simulink model "RADTRANS002"  (R2020b)
settings: Solver=VariableStepAuto  StartTime=0.0  StopTime=10.0  RelTol=1e-3
undefined symbols (not defined in the file): Line_110_C, Line_110_L, Line_110_R, Line_220_C, Line_220_L, Line_220_R, Line_35_C, Line_35_L, Line_35_R, Line_6_L, Line_6_R, Sys_f_Hz, Sys_V_net_kV, Tr_110_35_L_pu, Tr_110_35_R_pu, Tr_110_35_Sn_VA, Tr_110_35_V_HV_kV, Tr_110_35_V_LV_kV, Tr_110_6_L_pu, Tr_110_6_R_pu, Tr_110_6_Sn_VA, Tr_110_6_V_HV_kV, Tr_110_6_V_LV_kV, Tr_220_110_L_pu, Tr_220_110_R_pu, Tr_220_110_Sn_VA, Tr_220_110_V_HV_kV, Tr_220_110_V_LV_kV, Tr_35_04_L_pu, Tr_35_04_R_pu, Tr_35_04_Sn_VA, Tr_35_04_V_HV_kV, Tr_35_04_V_LV_kV, Tr_6_04_L_pu, Tr_6_04_R_pu, Tr_6_04_Sn_VA, Tr_6_04_V_HV_kV, Tr_6_04_V_LV_kV, Ts_powergui
libraries: dspstat3 x288, powerlib x202, powerlib_meascontrol x72
(part 3 of 7)

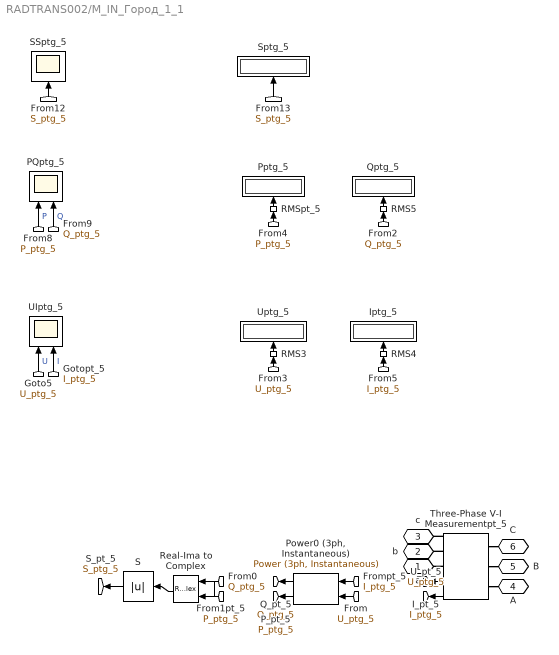
== system RADTRANS002/M_IN_Город_1_1 ==
  Iptg_5 : Display
      settings: Format=bank
  PQptg_5 : Scope  NumInputPorts=2
  "Power0 (3ph, Instantaneous)" : powerlib_meascontrol/Measurements/Power (3ph, Instantaneous)
  Pptg_5 : Display
      settings: Format=bank
  Qptg_5 : Display
      settings: Format=bank
  RMS3 : dspstat3/RMS  run=off  directionMode=Each column  dimension=1  InputProcessing=Columns as channels (frame based)  reset_popup=None
  RMS4 : dspstat3/RMS  run=off  directionMode=Each column  dimension=1  InputProcessing=Columns as channels (frame based)  reset_popup=None
  RMS5 : dspstat3/RMS  run=off  directionMode=Each column  dimension=1  InputProcessing=Columns as channels (frame based)  reset_popup=None
  RMSpt_5 : dspstat3/RMS  run=off  directionMode=Each column  dimension=1  InputProcessing=Columns as channels (frame based)  reset_popup=None
  Real-Ima to Complex : RealImagToComplex
  S : Abs
  SSptg_5 : Scope
  Sptg_5 : Display
      settings: Format=bank
  Three-Phase V-I Measurementpt_5 : powerlib/Measurements/Three-Phase V-I Measurement  VoltageMeasurement=phase-to-ground  SetLabelV=off  LabelV=Vabc  Vpu=off  VpuLL=off  CurrentMeasurement=yes  SetLabelI=off  LabelI=Iabc  Ipu=off  Pbase=100e6  Vbase=500e3  OutputType=Complex  PhasorSimulation=off  PSBequivalent=0
  UIptg_5 : Scope  NumInputPorts=2
  Uptg_5 : Display
      settings: Format=bank
  a : PMIOPort  Side=Right
  b : PMIOPort  Port=2  Side=Right
  c : PMIOPort  Port=3  Side=Right
  A : PMIOPort  Port=4  Side=Left
  B : PMIOPort  Port=5  Side=Left
  C : PMIOPort  Port=6  Side=Left
  tag scope: I_ptg_5=global, P_ptg_5=global, Q_ptg_5=global, S_ptg_5=global, U_ptg_5=global
  wires:
  S/1 -> [S_ptg_5]
  Real-Ima to Complex/1 -> S/1
  [S_ptg_5] -> Sptg_5/1
  [S_ptg_5] -> SSptg_5/1
  [P_ptg_5] -> RMSpt_5/1
  RMSpt_5/1 -> Pptg_5/1
  RMS5/1 -> Qptg_5/1
  [U_ptg_5] -> RMS3/1
  RMS3/1 -> Uptg_5/1
  [P_ptg_5] -> Real-Ima to Complex/1
  [Q_ptg_5] -> RMS5/1
  [I_ptg_5] -> RMS4/1
  RMS4/1 -> Iptg_5/1
  [U_ptg_5] -> UIptg_5/1  "U"
  [P_ptg_5] -> PQptg_5/1  "P"
  [I_ptg_5] -> UIptg_5/2  "I"
  Three-Phase V-I Measurementpt_5/1 -> [U_ptg_5]
  [Q_ptg_5] -> Real-Ima to Complex/2
  Three-Phase V-I Measurementpt_5/2 -> [I_ptg_5]
  [U_ptg_5] -> "Power0 (3ph, Instantaneous)"/1
  [I_ptg_5] -> "Power0 (3ph, Instantaneous)"/2
  "Power0 (3ph, Instantaneous)"/2 -> [Q_ptg_5]
  "Power0 (3ph, Instantaneous)"/1 -> [P_ptg_5]
  [Q_ptg_5] -> PQptg_5/2  "Q"
  connections:
  Three-Phase V-I Measurementpt_5/LConn1 -- A/RConn1
  Three-Phase V-I Measurementpt_5/RConn1 -- a/RConn1
  Three-Phase V-I Measurementpt_5/LConn2 -- B/RConn1
  Three-Phase V-I Measurementpt_5/LConn3 -- C/RConn1
  Three-Phase V-I Measurementpt_5/RConn3 -- c/RConn1
  Three-Phase V-I Measurementpt_5/RConn2 -- b/RConn1

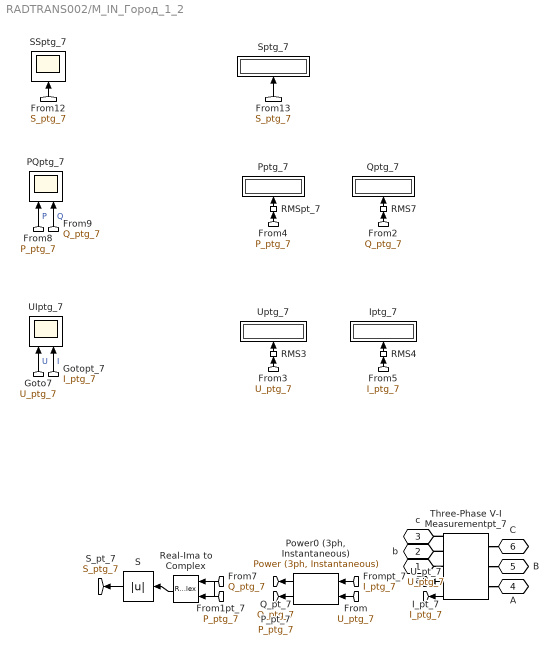
== system RADTRANS002/M_IN_Город_1_2 ==
  Iptg_7 : Display
      settings: Format=bank
  PQptg_7 : Scope  NumInputPorts=2
  "Power0 (3ph, Instantaneous)" : powerlib_meascontrol/Measurements/Power (3ph, Instantaneous)
  Pptg_7 : Display
      settings: Format=bank
  Qptg_7 : Display
      settings: Format=bank
  RMS3 : dspstat3/RMS  run=off  directionMode=Each column  dimension=1  InputProcessing=Columns as channels (frame based)  reset_popup=None
  RMS4 : dspstat3/RMS  run=off  directionMode=Each column  dimension=1  InputProcessing=Columns as channels (frame based)  reset_popup=None
  RMS7 : dspstat3/RMS  run=off  directionMode=Each column  dimension=1  InputProcessing=Columns as channels (frame based)  reset_popup=None
  RMSpt_7 : dspstat3/RMS  run=off  directionMode=Each column  dimension=1  InputProcessing=Columns as channels (frame based)  reset_popup=None
  Real-Ima to Complex : RealImagToComplex
  S : Abs
  SSptg_7 : Scope
  Sptg_7 : Display
      settings: Format=bank
  Three-Phase V-I Measurementpt_7 : powerlib/Measurements/Three-Phase V-I Measurement  VoltageMeasurement=phase-to-ground  SetLabelV=off  LabelV=Vabc  Vpu=off  VpuLL=off  CurrentMeasurement=yes  SetLabelI=off  LabelI=Iabc  Ipu=off  Pbase=100e6  Vbase=500e3  OutputType=Complex  PhasorSimulation=off  PSBequivalent=0
  UIptg_7 : Scope  NumInputPorts=2
  Uptg_7 : Display
      settings: Format=bank
  a : PMIOPort  Side=Right
  b : PMIOPort  Port=2  Side=Right
  c : PMIOPort  Port=3  Side=Right
  A : PMIOPort  Port=4  Side=Left
  B : PMIOPort  Port=5  Side=Left
  C : PMIOPort  Port=6  Side=Left
  tag scope: I_ptg_7=global, P_ptg_7=global, Q_ptg_7=global, S_ptg_7=global, U_ptg_7=global
  wires:
  S/1 -> [S_ptg_7]
  Real-Ima to Complex/1 -> S/1
  [S_ptg_7] -> Sptg_7/1
  [S_ptg_7] -> SSptg_7/1
  [P_ptg_7] -> RMSpt_7/1
  RMSpt_7/1 -> Pptg_7/1
  RMS7/1 -> Qptg_7/1
  [U_ptg_7] -> RMS3/1
  RMS3/1 -> Uptg_7/1
  [P_ptg_7] -> Real-Ima to Complex/1
  [Q_ptg_7] -> RMS7/1
  [I_ptg_7] -> RMS4/1
  RMS4/1 -> Iptg_7/1
  [U_ptg_7] -> UIptg_7/1  "U"
  [P_ptg_7] -> PQptg_7/1  "P"
  [I_ptg_7] -> UIptg_7/2  "I"
  Three-Phase V-I Measurementpt_7/1 -> [U_ptg_7]
  [Q_ptg_7] -> Real-Ima to Complex/2
  Three-Phase V-I Measurementpt_7/2 -> [I_ptg_7]
  [U_ptg_7] -> "Power0 (3ph, Instantaneous)"/1
  [I_ptg_7] -> "Power0 (3ph, Instantaneous)"/2
  "Power0 (3ph, Instantaneous)"/2 -> [Q_ptg_7]
  "Power0 (3ph, Instantaneous)"/1 -> [P_ptg_7]
  [Q_ptg_7] -> PQptg_7/2  "Q"
  connections:
  Three-Phase V-I Measurementpt_7/LConn1 -- A/RConn1
  Three-Phase V-I Measurementpt_7/RConn1 -- a/RConn1
  Three-Phase V-I Measurementpt_7/LConn2 -- B/RConn1
  Three-Phase V-I Measurementpt_7/LConn3 -- C/RConn1
  Three-Phase V-I Measurementpt_7/RConn3 -- c/RConn1
  Three-Phase V-I Measurementpt_7/RConn2 -- b/RConn1

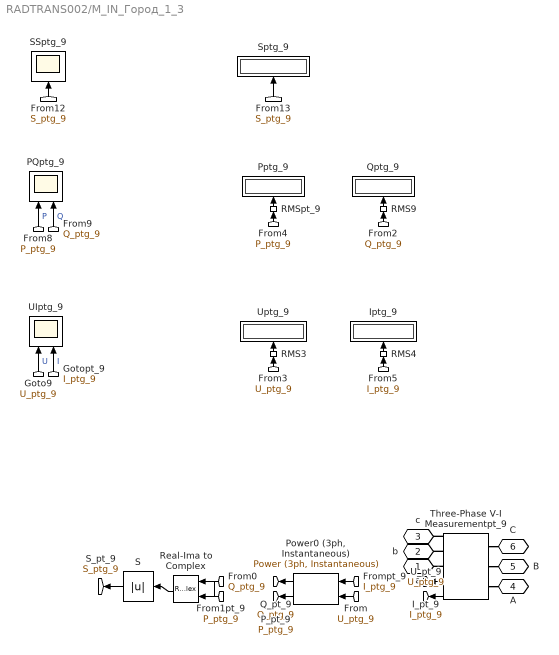
== system RADTRANS002/M_IN_Город_1_3 ==
  Iptg_9 : Display
      settings: Format=bank
  PQptg_9 : Scope  NumInputPorts=2
  "Power0 (3ph, Instantaneous)" : powerlib_meascontrol/Measurements/Power (3ph, Instantaneous)
  Pptg_9 : Display
      settings: Format=bank
  Qptg_9 : Display
      settings: Format=bank
  RMS3 : dspstat3/RMS  run=off  directionMode=Each column  dimension=1  InputProcessing=Columns as channels (frame based)  reset_popup=None
  RMS4 : dspstat3/RMS  run=off  directionMode=Each column  dimension=1  InputProcessing=Columns as channels (frame based)  reset_popup=None
  RMS9 : dspstat3/RMS  run=off  directionMode=Each column  dimension=1  InputProcessing=Columns as channels (frame based)  reset_popup=None
  RMSpt_9 : dspstat3/RMS  run=off  directionMode=Each column  dimension=1  InputProcessing=Columns as channels (frame based)  reset_popup=None
  Real-Ima to Complex : RealImagToComplex
  S : Abs
  SSptg_9 : Scope
  Sptg_9 : Display
      settings: Format=bank
  Three-Phase V-I Measurementpt_9 : powerlib/Measurements/Three-Phase V-I Measurement  VoltageMeasurement=phase-to-ground  SetLabelV=off  LabelV=Vabc  Vpu=off  VpuLL=off  CurrentMeasurement=yes  SetLabelI=off  LabelI=Iabc  Ipu=off  Pbase=100e6  Vbase=500e3  OutputType=Complex  PhasorSimulation=off  PSBequivalent=0
  UIptg_9 : Scope  NumInputPorts=2
  Uptg_9 : Display
      settings: Format=bank
  a : PMIOPort  Side=Right
  b : PMIOPort  Port=2  Side=Right
  c : PMIOPort  Port=3  Side=Right
  A : PMIOPort  Port=4  Side=Left
  B : PMIOPort  Port=5  Side=Left
  C : PMIOPort  Port=6  Side=Left
  tag scope: I_ptg_9=global, P_ptg_9=global, Q_ptg_9=global, S_ptg_9=global, U_ptg_9=global
  wires:
  S/1 -> [S_ptg_9]
  Real-Ima to Complex/1 -> S/1
  [S_ptg_9] -> Sptg_9/1
  [S_ptg_9] -> SSptg_9/1
  [P_ptg_9] -> RMSpt_9/1
  RMSpt_9/1 -> Pptg_9/1
  RMS9/1 -> Qptg_9/1
  [U_ptg_9] -> RMS3/1
  RMS3/1 -> Uptg_9/1
  [P_ptg_9] -> Real-Ima to Complex/1
  [Q_ptg_9] -> RMS9/1
  [I_ptg_9] -> RMS4/1
  RMS4/1 -> Iptg_9/1
  [U_ptg_9] -> UIptg_9/1  "U"
  [P_ptg_9] -> PQptg_9/1  "P"
  [I_ptg_9] -> UIptg_9/2  "I"
  Three-Phase V-I Measurementpt_9/1 -> [U_ptg_9]
  [Q_ptg_9] -> Real-Ima to Complex/2
  Three-Phase V-I Measurementpt_9/2 -> [I_ptg_9]
  [U_ptg_9] -> "Power0 (3ph, Instantaneous)"/1
  [I_ptg_9] -> "Power0 (3ph, Instantaneous)"/2
  "Power0 (3ph, Instantaneous)"/2 -> [Q_ptg_9]
  "Power0 (3ph, Instantaneous)"/1 -> [P_ptg_9]
  [Q_ptg_9] -> PQptg_9/2  "Q"
  connections:
  Three-Phase V-I Measurementpt_9/LConn1 -- A/RConn1
  Three-Phase V-I Measurementpt_9/RConn1 -- a/RConn1
  Three-Phase V-I Measurementpt_9/LConn2 -- B/RConn1
  Three-Phase V-I Measurementpt_9/LConn3 -- C/RConn1
  Three-Phase V-I Measurementpt_9/RConn3 -- c/RConn1
  Three-Phase V-I Measurementpt_9/RConn2 -- b/RConn1

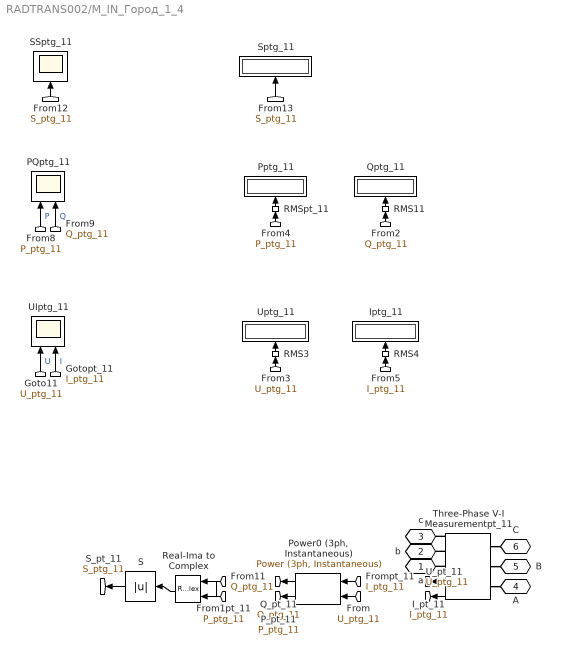
== system RADTRANS002/M_IN_Город_1_4 ==
  Iptg_11 : Display
      settings: Format=bank
  PQptg_11 : Scope  NumInputPorts=2
  "Power0 (3ph, Instantaneous)" : powerlib_meascontrol/Measurements/Power (3ph, Instantaneous)
  Pptg_11 : Display
      settings: Format=bank
  Qptg_11 : Display
      settings: Format=bank
  RMS11 : dspstat3/RMS  run=off  directionMode=Each column  dimension=1  InputProcessing=Columns as channels (frame based)  reset_popup=None
  RMS3 : dspstat3/RMS  run=off  directionMode=Each column  dimension=1  InputProcessing=Columns as channels (frame based)  reset_popup=None
  RMS4 : dspstat3/RMS  run=off  directionMode=Each column  dimension=1  InputProcessing=Columns as channels (frame based)  reset_popup=None
  RMSpt_11 : dspstat3/RMS  run=off  directionMode=Each column  dimension=1  InputProcessing=Columns as channels (frame based)  reset_popup=None
  Real-Ima to Complex : RealImagToComplex
  S : Abs
  SSptg_11 : Scope
  Sptg_11 : Display
      settings: Format=bank
  Three-Phase V-I Measurementpt_11 : powerlib/Measurements/Three-Phase V-I Measurement  VoltageMeasurement=phase-to-ground  SetLabelV=off  LabelV=Vabc  Vpu=off  VpuLL=off  CurrentMeasurement=yes  SetLabelI=off  LabelI=Iabc  Ipu=off  Pbase=100e6  Vbase=500e3  OutputType=Complex  PhasorSimulation=off  PSBequivalent=0
  UIptg_11 : Scope  NumInputPorts=2
  Uptg_11 : Display
      settings: Format=bank
  a : PMIOPort  Side=Right
  b : PMIOPort  Port=2  Side=Right
  c : PMIOPort  Port=3  Side=Right
  A : PMIOPort  Port=4  Side=Left
  B : PMIOPort  Port=5  Side=Left
  C : PMIOPort  Port=6  Side=Left
  tag scope: I_ptg_11=global, P_ptg_11=global, Q_ptg_11=global, S_ptg_11=global, U_ptg_11=global
  wires:
  S/1 -> [S_ptg_11]
  Real-Ima to Complex/1 -> S/1
  [S_ptg_11] -> Sptg_11/1
  [S_ptg_11] -> SSptg_11/1
  [P_ptg_11] -> RMSpt_11/1
  RMSpt_11/1 -> Pptg_11/1
  RMS11/1 -> Qptg_11/1
  [U_ptg_11] -> RMS3/1
  RMS3/1 -> Uptg_11/1
  [P_ptg_11] -> Real-Ima to Complex/1
  [Q_ptg_11] -> RMS11/1
  [I_ptg_11] -> RMS4/1
  RMS4/1 -> Iptg_11/1
  [U_ptg_11] -> UIptg_11/1  "U"
  [P_ptg_11] -> PQptg_11/1  "P"
  [I_ptg_11] -> UIptg_11/2  "I"
  Three-Phase V-I Measurementpt_11/1 -> [U_ptg_11]
  [Q_ptg_11] -> Real-Ima to Complex/2
  Three-Phase V-I Measurementpt_11/2 -> [I_ptg_11]
  [U_ptg_11] -> "Power0 (3ph, Instantaneous)"/1
  [I_ptg_11] -> "Power0 (3ph, Instantaneous)"/2
  "Power0 (3ph, Instantaneous)"/2 -> [Q_ptg_11]
  "Power0 (3ph, Instantaneous)"/1 -> [P_ptg_11]
  [Q_ptg_11] -> PQptg_11/2  "Q"
  connections:
  Three-Phase V-I Measurementpt_11/LConn1 -- A/RConn1
  Three-Phase V-I Measurementpt_11/RConn1 -- a/RConn1
  Three-Phase V-I Measurementpt_11/LConn2 -- B/RConn1
  Three-Phase V-I Measurementpt_11/LConn3 -- C/RConn1
  Three-Phase V-I Measurementpt_11/RConn3 -- c/RConn1
  Three-Phase V-I Measurementpt_11/RConn2 -- b/RConn1

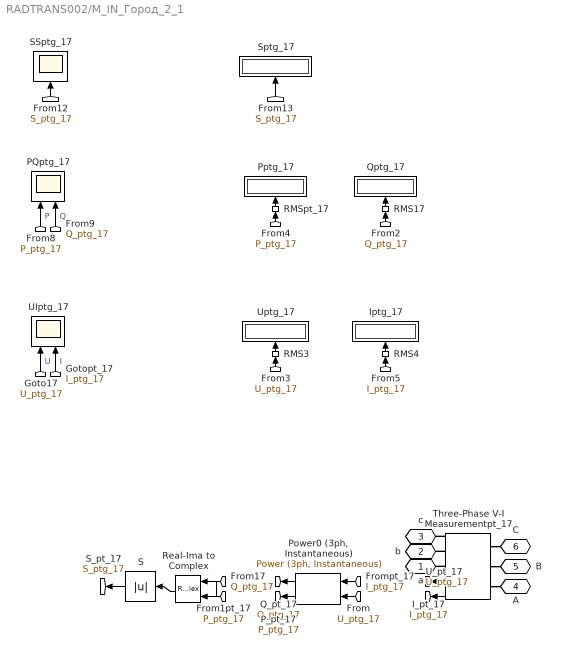
== system RADTRANS002/M_IN_Город_2_1 ==
  Iptg_17 : Display
      settings: Format=bank
  PQptg_17 : Scope  NumInputPorts=2
  "Power0 (3ph, Instantaneous)" : powerlib_meascontrol/Measurements/Power (3ph, Instantaneous)
  Pptg_17 : Display
      settings: Format=bank
  Qptg_17 : Display
      settings: Format=bank
  RMS17 : dspstat3/RMS  run=off  directionMode=Each column  dimension=1  InputProcessing=Columns as channels (frame based)  reset_popup=None
  RMS3 : dspstat3/RMS  run=off  directionMode=Each column  dimension=1  InputProcessing=Columns as channels (frame based)  reset_popup=None
  RMS4 : dspstat3/RMS  run=off  directionMode=Each column  dimension=1  InputProcessing=Columns as channels (frame based)  reset_popup=None
  RMSpt_17 : dspstat3/RMS  run=off  directionMode=Each column  dimension=1  InputProcessing=Columns as channels (frame based)  reset_popup=None
  Real-Ima to Complex : RealImagToComplex
  S : Abs
  SSptg_17 : Scope
  Sptg_17 : Display
      settings: Format=bank
  Three-Phase V-I Measurementpt_17 : powerlib/Measurements/Three-Phase V-I Measurement  VoltageMeasurement=phase-to-ground  SetLabelV=off  LabelV=Vabc  Vpu=off  VpuLL=off  CurrentMeasurement=yes  SetLabelI=off  LabelI=Iabc  Ipu=off  Pbase=100e6  Vbase=500e3  OutputType=Complex  PhasorSimulation=off  PSBequivalent=0
  UIptg_17 : Scope  NumInputPorts=2
  Uptg_17 : Display
      settings: Format=bank
  a : PMIOPort  Side=Right
  b : PMIOPort  Port=2  Side=Right
  c : PMIOPort  Port=3  Side=Right
  A : PMIOPort  Port=4  Side=Left
  B : PMIOPort  Port=5  Side=Left
  C : PMIOPort  Port=6  Side=Left
  tag scope: I_ptg_17=global, P_ptg_17=global, Q_ptg_17=global, S_ptg_17=global, U_ptg_17=global
  wires:
  S/1 -> [S_ptg_17]
  Real-Ima to Complex/1 -> S/1
  [S_ptg_17] -> Sptg_17/1
  [S_ptg_17] -> SSptg_17/1
  [P_ptg_17] -> RMSpt_17/1
  RMSpt_17/1 -> Pptg_17/1
  RMS17/1 -> Qptg_17/1
  [U_ptg_17] -> RMS3/1
  RMS3/1 -> Uptg_17/1
  [P_ptg_17] -> Real-Ima to Complex/1
  [Q_ptg_17] -> RMS17/1
  [I_ptg_17] -> RMS4/1
  RMS4/1 -> Iptg_17/1
  [U_ptg_17] -> UIptg_17/1  "U"
  [P_ptg_17] -> PQptg_17/1  "P"
  [I_ptg_17] -> UIptg_17/2  "I"
  Three-Phase V-I Measurementpt_17/1 -> [U_ptg_17]
  [Q_ptg_17] -> Real-Ima to Complex/2
  Three-Phase V-I Measurementpt_17/2 -> [I_ptg_17]
  [U_ptg_17] -> "Power0 (3ph, Instantaneous)"/1
  [I_ptg_17] -> "Power0 (3ph, Instantaneous)"/2
  "Power0 (3ph, Instantaneous)"/2 -> [Q_ptg_17]
  "Power0 (3ph, Instantaneous)"/1 -> [P_ptg_17]
  [Q_ptg_17] -> PQptg_17/2  "Q"
  connections:
  Three-Phase V-I Measurementpt_17/LConn1 -- A/RConn1
  Three-Phase V-I Measurementpt_17/RConn1 -- a/RConn1
  Three-Phase V-I Measurementpt_17/LConn2 -- B/RConn1
  Three-Phase V-I Measurementpt_17/LConn3 -- C/RConn1
  Three-Phase V-I Measurementpt_17/RConn3 -- c/RConn1
  Three-Phase V-I Measurementpt_17/RConn2 -- b/RConn1

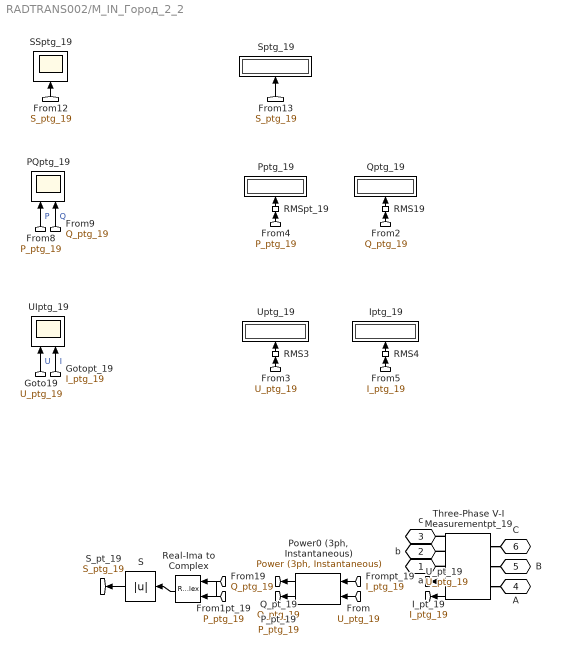
== system RADTRANS002/M_IN_Город_2_2 ==
  Iptg_19 : Display
      settings: Format=bank
  PQptg_19 : Scope  NumInputPorts=2
  "Power0 (3ph, Instantaneous)" : powerlib_meascontrol/Measurements/Power (3ph, Instantaneous)
  Pptg_19 : Display
      settings: Format=bank
  Qptg_19 : Display
      settings: Format=bank
  RMS19 : dspstat3/RMS  run=off  directionMode=Each column  dimension=1  InputProcessing=Columns as channels (frame based)  reset_popup=None
  RMS3 : dspstat3/RMS  run=off  directionMode=Each column  dimension=1  InputProcessing=Columns as channels (frame based)  reset_popup=None
  RMS4 : dspstat3/RMS  run=off  directionMode=Each column  dimension=1  InputProcessing=Columns as channels (frame based)  reset_popup=None
  RMSpt_19 : dspstat3/RMS  run=off  directionMode=Each column  dimension=1  InputProcessing=Columns as channels (frame based)  reset_popup=None
  Real-Ima to Complex : RealImagToComplex
  S : Abs
  SSptg_19 : Scope
  Sptg_19 : Display
      settings: Format=bank
  Three-Phase V-I Measurementpt_19 : powerlib/Measurements/Three-Phase V-I Measurement  VoltageMeasurement=phase-to-ground  SetLabelV=off  LabelV=Vabc  Vpu=off  VpuLL=off  CurrentMeasurement=yes  SetLabelI=off  LabelI=Iabc  Ipu=off  Pbase=100e6  Vbase=500e3  OutputType=Complex  PhasorSimulation=off  PSBequivalent=0
  UIptg_19 : Scope  NumInputPorts=2
  Uptg_19 : Display
      settings: Format=bank
  a : PMIOPort  Side=Right
  b : PMIOPort  Port=2  Side=Right
  c : PMIOPort  Port=3  Side=Right
  A : PMIOPort  Port=4  Side=Left
  B : PMIOPort  Port=5  Side=Left
  C : PMIOPort  Port=6  Side=Left
  tag scope: I_ptg_19=global, P_ptg_19=global, Q_ptg_19=global, S_ptg_19=global, U_ptg_19=global
  wires:
  S/1 -> [S_ptg_19]
  Real-Ima to Complex/1 -> S/1
  [S_ptg_19] -> Sptg_19/1
  [S_ptg_19] -> SSptg_19/1
  [P_ptg_19] -> RMSpt_19/1
  RMSpt_19/1 -> Pptg_19/1
  RMS19/1 -> Qptg_19/1
  [U_ptg_19] -> RMS3/1
  RMS3/1 -> Uptg_19/1
  [P_ptg_19] -> Real-Ima to Complex/1
  [Q_ptg_19] -> RMS19/1
  [I_ptg_19] -> RMS4/1
  RMS4/1 -> Iptg_19/1
  [U_ptg_19] -> UIptg_19/1  "U"
  [P_ptg_19] -> PQptg_19/1  "P"
  [I_ptg_19] -> UIptg_19/2  "I"
  Three-Phase V-I Measurementpt_19/1 -> [U_ptg_19]
  [Q_ptg_19] -> Real-Ima to Complex/2
  Three-Phase V-I Measurementpt_19/2 -> [I_ptg_19]
  [U_ptg_19] -> "Power0 (3ph, Instantaneous)"/1
  [I_ptg_19] -> "Power0 (3ph, Instantaneous)"/2
  "Power0 (3ph, Instantaneous)"/2 -> [Q_ptg_19]
  "Power0 (3ph, Instantaneous)"/1 -> [P_ptg_19]
  [Q_ptg_19] -> PQptg_19/2  "Q"
  connections:
  Three-Phase V-I Measurementpt_19/LConn1 -- A/RConn1
  Three-Phase V-I Measurementpt_19/RConn1 -- a/RConn1
  Three-Phase V-I Measurementpt_19/LConn2 -- B/RConn1
  Three-Phase V-I Measurementpt_19/LConn3 -- C/RConn1
  Three-Phase V-I Measurementpt_19/RConn3 -- c/RConn1
  Three-Phase V-I Measurementpt_19/RConn2 -- b/RConn1

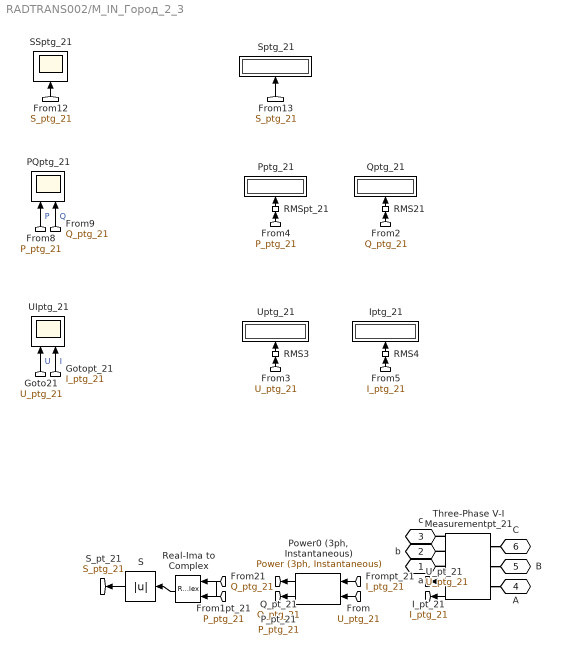
== system RADTRANS002/M_IN_Город_2_3 ==
  Iptg_21 : Display
      settings: Format=bank
  PQptg_21 : Scope  NumInputPorts=2
  "Power0 (3ph, Instantaneous)" : powerlib_meascontrol/Measurements/Power (3ph, Instantaneous)
  Pptg_21 : Display
      settings: Format=bank
  Qptg_21 : Display
      settings: Format=bank
  RMS21 : dspstat3/RMS  run=off  directionMode=Each column  dimension=1  InputProcessing=Columns as channels (frame based)  reset_popup=None
  RMS3 : dspstat3/RMS  run=off  directionMode=Each column  dimension=1  InputProcessing=Columns as channels (frame based)  reset_popup=None
  RMS4 : dspstat3/RMS  run=off  directionMode=Each column  dimension=1  InputProcessing=Columns as channels (frame based)  reset_popup=None
  RMSpt_21 : dspstat3/RMS  run=off  directionMode=Each column  dimension=1  InputProcessing=Columns as channels (frame based)  reset_popup=None
  Real-Ima to Complex : RealImagToComplex
  S : Abs
  SSptg_21 : Scope
  Sptg_21 : Display
      settings: Format=bank
  Three-Phase V-I Measurementpt_21 : powerlib/Measurements/Three-Phase V-I Measurement  VoltageMeasurement=phase-to-ground  SetLabelV=off  LabelV=Vabc  Vpu=off  VpuLL=off  CurrentMeasurement=yes  SetLabelI=off  LabelI=Iabc  Ipu=off  Pbase=100e6  Vbase=500e3  OutputType=Complex  PhasorSimulation=off  PSBequivalent=0
  UIptg_21 : Scope  NumInputPorts=2
  Uptg_21 : Display
      settings: Format=bank
  a : PMIOPort  Side=Right
  b : PMIOPort  Port=2  Side=Right
  c : PMIOPort  Port=3  Side=Right
  A : PMIOPort  Port=4  Side=Left
  B : PMIOPort  Port=5  Side=Left
  C : PMIOPort  Port=6  Side=Left
  tag scope: I_ptg_21=global, P_ptg_21=global, Q_ptg_21=global, S_ptg_21=global, U_ptg_21=global
  wires:
  S/1 -> [S_ptg_21]
  Real-Ima to Complex/1 -> S/1
  [S_ptg_21] -> Sptg_21/1
  [S_ptg_21] -> SSptg_21/1
  [P_ptg_21] -> RMSpt_21/1
  RMSpt_21/1 -> Pptg_21/1
  RMS21/1 -> Qptg_21/1
  [U_ptg_21] -> RMS3/1
  RMS3/1 -> Uptg_21/1
  [P_ptg_21] -> Real-Ima to Complex/1
  [Q_ptg_21] -> RMS21/1
  [I_ptg_21] -> RMS4/1
  RMS4/1 -> Iptg_21/1
  [U_ptg_21] -> UIptg_21/1  "U"
  [P_ptg_21] -> PQptg_21/1  "P"
  [I_ptg_21] -> UIptg_21/2  "I"
  Three-Phase V-I Measurementpt_21/1 -> [U_ptg_21]
  [Q_ptg_21] -> Real-Ima to Complex/2
  Three-Phase V-I Measurementpt_21/2 -> [I_ptg_21]
  [U_ptg_21] -> "Power0 (3ph, Instantaneous)"/1
  [I_ptg_21] -> "Power0 (3ph, Instantaneous)"/2
  "Power0 (3ph, Instantaneous)"/2 -> [Q_ptg_21]
  "Power0 (3ph, Instantaneous)"/1 -> [P_ptg_21]
  [Q_ptg_21] -> PQptg_21/2  "Q"
  connections:
  Three-Phase V-I Measurementpt_21/LConn1 -- A/RConn1
  Three-Phase V-I Measurementpt_21/RConn1 -- a/RConn1
  Three-Phase V-I Measurementpt_21/LConn2 -- B/RConn1
  Three-Phase V-I Measurementpt_21/LConn3 -- C/RConn1
  Three-Phase V-I Measurementpt_21/RConn3 -- c/RConn1
  Three-Phase V-I Measurementpt_21/RConn2 -- b/RConn1

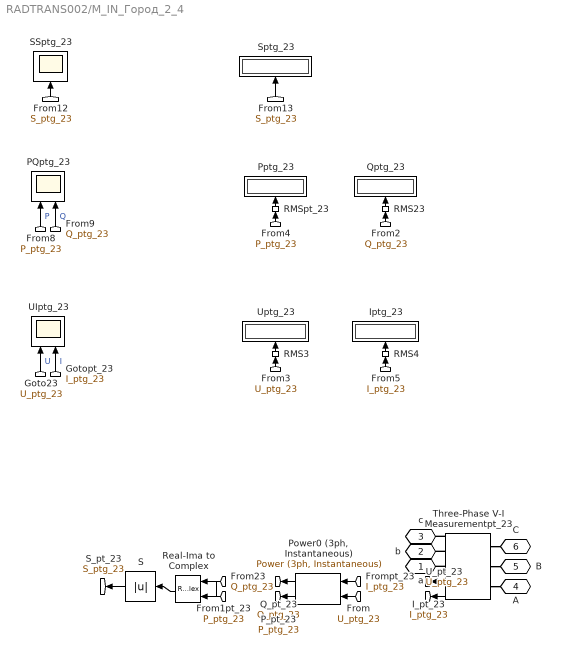
== system RADTRANS002/M_IN_Город_2_4 ==
  Iptg_23 : Display
      settings: Format=bank
  PQptg_23 : Scope  NumInputPorts=2
  "Power0 (3ph, Instantaneous)" : powerlib_meascontrol/Measurements/Power (3ph, Instantaneous)
  Pptg_23 : Display
      settings: Format=bank
  Qptg_23 : Display
      settings: Format=bank
  RMS23 : dspstat3/RMS  run=off  directionMode=Each column  dimension=1  InputProcessing=Columns as channels (frame based)  reset_popup=None
  RMS3 : dspstat3/RMS  run=off  directionMode=Each column  dimension=1  InputProcessing=Columns as channels (frame based)  reset_popup=None
  RMS4 : dspstat3/RMS  run=off  directionMode=Each column  dimension=1  InputProcessing=Columns as channels (frame based)  reset_popup=None
  RMSpt_23 : dspstat3/RMS  run=off  directionMode=Each column  dimension=1  InputProcessing=Columns as channels (frame based)  reset_popup=None
  Real-Ima to Complex : RealImagToComplex
  S : Abs
  SSptg_23 : Scope
  Sptg_23 : Display
      settings: Format=bank
  Three-Phase V-I Measurementpt_23 : powerlib/Measurements/Three-Phase V-I Measurement  VoltageMeasurement=phase-to-ground  SetLabelV=off  LabelV=Vabc  Vpu=off  VpuLL=off  CurrentMeasurement=yes  SetLabelI=off  LabelI=Iabc  Ipu=off  Pbase=100e6  Vbase=500e3  OutputType=Complex  PhasorSimulation=off  PSBequivalent=0
  UIptg_23 : Scope  NumInputPorts=2
  Uptg_23 : Display
      settings: Format=bank
  a : PMIOPort  Side=Right
  b : PMIOPort  Port=2  Side=Right
  c : PMIOPort  Port=3  Side=Right
  A : PMIOPort  Port=4  Side=Left
  B : PMIOPort  Port=5  Side=Left
  C : PMIOPort  Port=6  Side=Left
  tag scope: I_ptg_23=global, P_ptg_23=global, Q_ptg_23=global, S_ptg_23=global, U_ptg_23=global
  wires:
  S/1 -> [S_ptg_23]
  Real-Ima to Complex/1 -> S/1
  [S_ptg_23] -> Sptg_23/1
  [S_ptg_23] -> SSptg_23/1
  [P_ptg_23] -> RMSpt_23/1
  RMSpt_23/1 -> Pptg_23/1
  RMS23/1 -> Qptg_23/1
  [U_ptg_23] -> RMS3/1
  RMS3/1 -> Uptg_23/1
  [P_ptg_23] -> Real-Ima to Complex/1
  [Q_ptg_23] -> RMS23/1
  [I_ptg_23] -> RMS4/1
  RMS4/1 -> Iptg_23/1
  [U_ptg_23] -> UIptg_23/1  "U"
  [P_ptg_23] -> PQptg_23/1  "P"
  [I_ptg_23] -> UIptg_23/2  "I"
  Three-Phase V-I Measurementpt_23/1 -> [U_ptg_23]
  [Q_ptg_23] -> Real-Ima to Complex/2
  Three-Phase V-I Measurementpt_23/2 -> [I_ptg_23]
  [U_ptg_23] -> "Power0 (3ph, Instantaneous)"/1
  [I_ptg_23] -> "Power0 (3ph, Instantaneous)"/2
  "Power0 (3ph, Instantaneous)"/2 -> [Q_ptg_23]
  "Power0 (3ph, Instantaneous)"/1 -> [P_ptg_23]
  [Q_ptg_23] -> PQptg_23/2  "Q"
  connections:
  Three-Phase V-I Measurementpt_23/LConn1 -- A/RConn1
  Three-Phase V-I Measurementpt_23/RConn1 -- a/RConn1
  Three-Phase V-I Measurementpt_23/LConn2 -- B/RConn1
  Three-Phase V-I Measurementpt_23/LConn3 -- C/RConn1
  Three-Phase V-I Measurementpt_23/RConn3 -- c/RConn1
  Three-Phase V-I Measurementpt_23/RConn2 -- b/RConn1

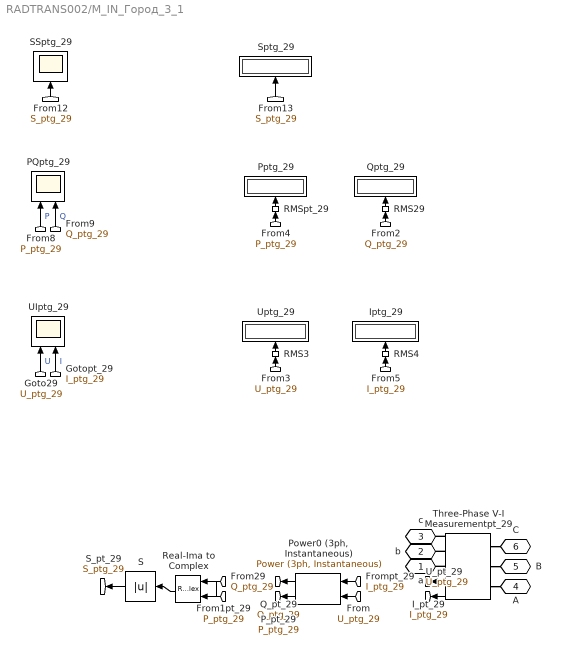
== system RADTRANS002/M_IN_Город_3_1 ==
  Iptg_29 : Display
      settings: Format=bank
  PQptg_29 : Scope  NumInputPorts=2
  "Power0 (3ph, Instantaneous)" : powerlib_meascontrol/Measurements/Power (3ph, Instantaneous)
  Pptg_29 : Display
      settings: Format=bank
  Qptg_29 : Display
      settings: Format=bank
  RMS29 : dspstat3/RMS  run=off  directionMode=Each column  dimension=1  InputProcessing=Columns as channels (frame based)  reset_popup=None
  RMS3 : dspstat3/RMS  run=off  directionMode=Each column  dimension=1  InputProcessing=Columns as channels (frame based)  reset_popup=None
  RMS4 : dspstat3/RMS  run=off  directionMode=Each column  dimension=1  InputProcessing=Columns as channels (frame based)  reset_popup=None
  RMSpt_29 : dspstat3/RMS  run=off  directionMode=Each column  dimension=1  InputProcessing=Columns as channels (frame based)  reset_popup=None
  Real-Ima to Complex : RealImagToComplex
  S : Abs
  SSptg_29 : Scope
  Sptg_29 : Display
      settings: Format=bank
  Three-Phase V-I Measurementpt_29 : powerlib/Measurements/Three-Phase V-I Measurement  VoltageMeasurement=phase-to-ground  SetLabelV=off  LabelV=Vabc  Vpu=off  VpuLL=off  CurrentMeasurement=yes  SetLabelI=off  LabelI=Iabc  Ipu=off  Pbase=100e6  Vbase=500e3  OutputType=Complex  PhasorSimulation=off  PSBequivalent=0
  UIptg_29 : Scope  NumInputPorts=2
  Uptg_29 : Display
      settings: Format=bank
  a : PMIOPort  Side=Right
  b : PMIOPort  Port=2  Side=Right
  c : PMIOPort  Port=3  Side=Right
  A : PMIOPort  Port=4  Side=Left
  B : PMIOPort  Port=5  Side=Left
  C : PMIOPort  Port=6  Side=Left
  tag scope: I_ptg_29=global, P_ptg_29=global, Q_ptg_29=global, S_ptg_29=global, U_ptg_29=global
  wires:
  S/1 -> [S_ptg_29]
  Real-Ima to Complex/1 -> S/1
  [S_ptg_29] -> Sptg_29/1
  [S_ptg_29] -> SSptg_29/1
  [P_ptg_29] -> RMSpt_29/1
  RMSpt_29/1 -> Pptg_29/1
  RMS29/1 -> Qptg_29/1
  [U_ptg_29] -> RMS3/1
  RMS3/1 -> Uptg_29/1
  [P_ptg_29] -> Real-Ima to Complex/1
  [Q_ptg_29] -> RMS29/1
  [I_ptg_29] -> RMS4/1
  RMS4/1 -> Iptg_29/1
  [U_ptg_29] -> UIptg_29/1  "U"
  [P_ptg_29] -> PQptg_29/1  "P"
  [I_ptg_29] -> UIptg_29/2  "I"
  Three-Phase V-I Measurementpt_29/1 -> [U_ptg_29]
  [Q_ptg_29] -> Real-Ima to Complex/2
  Three-Phase V-I Measurementpt_29/2 -> [I_ptg_29]
  [U_ptg_29] -> "Power0 (3ph, Instantaneous)"/1
  [I_ptg_29] -> "Power0 (3ph, Instantaneous)"/2
  "Power0 (3ph, Instantaneous)"/2 -> [Q_ptg_29]
  "Power0 (3ph, Instantaneous)"/1 -> [P_ptg_29]
  [Q_ptg_29] -> PQptg_29/2  "Q"
  connections:
  Three-Phase V-I Measurementpt_29/LConn1 -- A/RConn1
  Three-Phase V-I Measurementpt_29/RConn1 -- a/RConn1
  Three-Phase V-I Measurementpt_29/LConn2 -- B/RConn1
  Three-Phase V-I Measurementpt_29/LConn3 -- C/RConn1
  Three-Phase V-I Measurementpt_29/RConn3 -- c/RConn1
  Three-Phase V-I Measurementpt_29/RConn2 -- b/RConn1

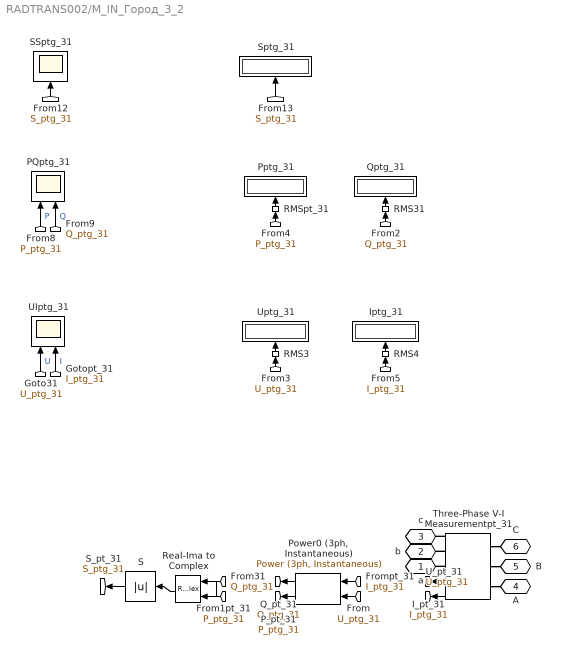
== system RADTRANS002/M_IN_Город_3_2 ==
  Iptg_31 : Display
      settings: Format=bank
  PQptg_31 : Scope  NumInputPorts=2
  "Power0 (3ph, Instantaneous)" : powerlib_meascontrol/Measurements/Power (3ph, Instantaneous)
  Pptg_31 : Display
      settings: Format=bank
  Qptg_31 : Display
      settings: Format=bank
  RMS3 : dspstat3/RMS  run=off  directionMode=Each column  dimension=1  InputProcessing=Columns as channels (frame based)  reset_popup=None
  RMS31 : dspstat3/RMS  run=off  directionMode=Each column  dimension=1  InputProcessing=Columns as channels (frame based)  reset_popup=None
  RMS4 : dspstat3/RMS  run=off  directionMode=Each column  dimension=1  InputProcessing=Columns as channels (frame based)  reset_popup=None
  RMSpt_31 : dspstat3/RMS  run=off  directionMode=Each column  dimension=1  InputProcessing=Columns as channels (frame based)  reset_popup=None
  Real-Ima to Complex : RealImagToComplex
  S : Abs
  SSptg_31 : Scope
  Sptg_31 : Display
      settings: Format=bank
  Three-Phase V-I Measurementpt_31 : powerlib/Measurements/Three-Phase V-I Measurement  VoltageMeasurement=phase-to-ground  SetLabelV=off  LabelV=Vabc  Vpu=off  VpuLL=off  CurrentMeasurement=yes  SetLabelI=off  LabelI=Iabc  Ipu=off  Pbase=100e6  Vbase=500e3  OutputType=Complex  PhasorSimulation=off  PSBequivalent=0
  UIptg_31 : Scope  NumInputPorts=2
  Uptg_31 : Display
      settings: Format=bank
  a : PMIOPort  Side=Right
  b : PMIOPort  Port=2  Side=Right
  c : PMIOPort  Port=3  Side=Right
  A : PMIOPort  Port=4  Side=Left
  B : PMIOPort  Port=5  Side=Left
  C : PMIOPort  Port=6  Side=Left
  tag scope: I_ptg_31=global, P_ptg_31=global, Q_ptg_31=global, S_ptg_31=global, U_ptg_31=global
  wires:
  S/1 -> [S_ptg_31]
  Real-Ima to Complex/1 -> S/1
  [S_ptg_31] -> Sptg_31/1
  [S_ptg_31] -> SSptg_31/1
  [P_ptg_31] -> RMSpt_31/1
  RMSpt_31/1 -> Pptg_31/1
  RMS31/1 -> Qptg_31/1
  [U_ptg_31] -> RMS3/1
  RMS3/1 -> Uptg_31/1
  [P_ptg_31] -> Real-Ima to Complex/1
  [Q_ptg_31] -> RMS31/1
  [I_ptg_31] -> RMS4/1
  RMS4/1 -> Iptg_31/1
  [U_ptg_31] -> UIptg_31/1  "U"
  [P_ptg_31] -> PQptg_31/1  "P"
  [I_ptg_31] -> UIptg_31/2  "I"
  Three-Phase V-I Measurementpt_31/1 -> [U_ptg_31]
  [Q_ptg_31] -> Real-Ima to Complex/2
  Three-Phase V-I Measurementpt_31/2 -> [I_ptg_31]
  [U_ptg_31] -> "Power0 (3ph, Instantaneous)"/1
  [I_ptg_31] -> "Power0 (3ph, Instantaneous)"/2
  "Power0 (3ph, Instantaneous)"/2 -> [Q_ptg_31]
  "Power0 (3ph, Instantaneous)"/1 -> [P_ptg_31]
  [Q_ptg_31] -> PQptg_31/2  "Q"
  connections:
  Three-Phase V-I Measurementpt_31/LConn1 -- A/RConn1
  Three-Phase V-I Measurementpt_31/RConn1 -- a/RConn1
  Three-Phase V-I Measurementpt_31/LConn2 -- B/RConn1
  Three-Phase V-I Measurementpt_31/LConn3 -- C/RConn1
  Three-Phase V-I Measurementpt_31/RConn3 -- c/RConn1
  Three-Phase V-I Measurementpt_31/RConn2 -- b/RConn1

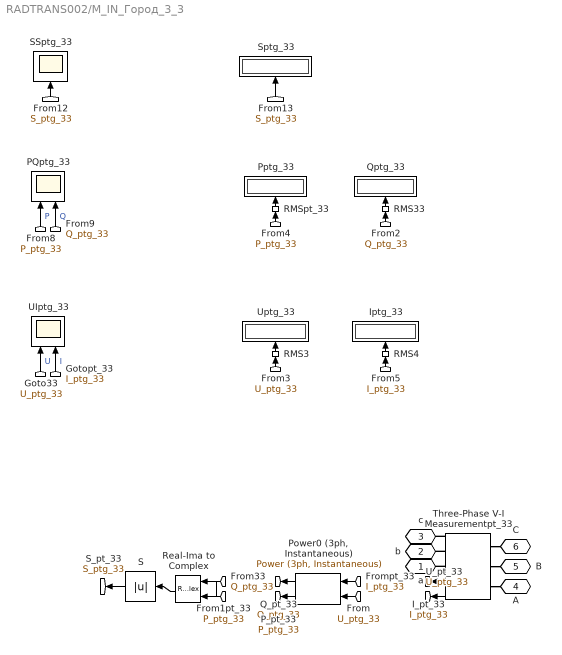
== system RADTRANS002/M_IN_Город_3_3 ==
  Iptg_33 : Display
      settings: Format=bank
  PQptg_33 : Scope  NumInputPorts=2
  "Power0 (3ph, Instantaneous)" : powerlib_meascontrol/Measurements/Power (3ph, Instantaneous)
  Pptg_33 : Display
      settings: Format=bank
  Qptg_33 : Display
      settings: Format=bank
  RMS3 : dspstat3/RMS  run=off  directionMode=Each column  dimension=1  InputProcessing=Columns as channels (frame based)  reset_popup=None
  RMS33 : dspstat3/RMS  run=off  directionMode=Each column  dimension=1  InputProcessing=Columns as channels (frame based)  reset_popup=None
  RMS4 : dspstat3/RMS  run=off  directionMode=Each column  dimension=1  InputProcessing=Columns as channels (frame based)  reset_popup=None
  RMSpt_33 : dspstat3/RMS  run=off  directionMode=Each column  dimension=1  InputProcessing=Columns as channels (frame based)  reset_popup=None
  Real-Ima to Complex : RealImagToComplex
  S : Abs
  SSptg_33 : Scope
  Sptg_33 : Display
      settings: Format=bank
  Three-Phase V-I Measurementpt_33 : powerlib/Measurements/Three-Phase V-I Measurement  VoltageMeasurement=phase-to-ground  SetLabelV=off  LabelV=Vabc  Vpu=off  VpuLL=off  CurrentMeasurement=yes  SetLabelI=off  LabelI=Iabc  Ipu=off  Pbase=100e6  Vbase=500e3  OutputType=Complex  PhasorSimulation=off  PSBequivalent=0
  UIptg_33 : Scope  NumInputPorts=2
  Uptg_33 : Display
      settings: Format=bank
  a : PMIOPort  Side=Right
  b : PMIOPort  Port=2  Side=Right
  c : PMIOPort  Port=3  Side=Right
  A : PMIOPort  Port=4  Side=Left
  B : PMIOPort  Port=5  Side=Left
  C : PMIOPort  Port=6  Side=Left
  tag scope: I_ptg_33=global, P_ptg_33=global, Q_ptg_33=global, S_ptg_33=global, U_ptg_33=global
  wires:
  S/1 -> [S_ptg_33]
  Real-Ima to Complex/1 -> S/1
  [S_ptg_33] -> Sptg_33/1
  [S_ptg_33] -> SSptg_33/1
  [P_ptg_33] -> RMSpt_33/1
  RMSpt_33/1 -> Pptg_33/1
  RMS33/1 -> Qptg_33/1
  [U_ptg_33] -> RMS3/1
  RMS3/1 -> Uptg_33/1
  [P_ptg_33] -> Real-Ima to Complex/1
  [Q_ptg_33] -> RMS33/1
  [I_ptg_33] -> RMS4/1
  RMS4/1 -> Iptg_33/1
  [U_ptg_33] -> UIptg_33/1  "U"
  [P_ptg_33] -> PQptg_33/1  "P"
  [I_ptg_33] -> UIptg_33/2  "I"
  Three-Phase V-I Measurementpt_33/1 -> [U_ptg_33]
  [Q_ptg_33] -> Real-Ima to Complex/2
  Three-Phase V-I Measurementpt_33/2 -> [I_ptg_33]
  [U_ptg_33] -> "Power0 (3ph, Instantaneous)"/1
  [I_ptg_33] -> "Power0 (3ph, Instantaneous)"/2
  "Power0 (3ph, Instantaneous)"/2 -> [Q_ptg_33]
  "Power0 (3ph, Instantaneous)"/1 -> [P_ptg_33]
  [Q_ptg_33] -> PQptg_33/2  "Q"
  connections:
  Three-Phase V-I Measurementpt_33/LConn1 -- A/RConn1
  Three-Phase V-I Measurementpt_33/RConn1 -- a/RConn1
  Three-Phase V-I Measurementpt_33/LConn2 -- B/RConn1
  Three-Phase V-I Measurementpt_33/LConn3 -- C/RConn1
  Three-Phase V-I Measurementpt_33/RConn3 -- c/RConn1
  Three-Phase V-I Measurementpt_33/RConn2 -- b/RConn1

== system RADTRANS002/M_IN_Город_3_4 ==
  Iptg_35 : Display
      settings: Format=bank
  PQptg_35 : Scope  NumInputPorts=2
  "Power0 (3ph, Instantaneous)" : powerlib_meascontrol/Measurements/Power (3ph, Instantaneous)
  Pptg_35 : Display
      settings: Format=bank
  Qptg_35 : Display
      settings: Format=bank
  RMS3 : dspstat3/RMS  run=off  directionMode=Each column  dimension=1  InputProcessing=Columns as channels (frame based)  reset_popup=None
  RMS35 : dspstat3/RMS  run=off  directionMode=Each column  dimension=1  InputProcessing=Columns as channels (frame based)  reset_popup=None
  RMS4 : dspstat3/RMS  run=off  directionMode=Each column  dimension=1  InputProcessing=Columns as channels (frame based)  reset_popup=None
  RMSpt_35 : dspstat3/RMS  run=off  directionMode=Each column  dimension=1  InputProcessing=Columns as channels (frame based)  reset_popup=None
  Real-Ima to Complex : RealImagToComplex
  S : Abs
  SSptg_35 : Scope
  Sptg_35 : Display
      settings: Format=bank
  Three-Phase V-I Measurementpt_35 : powerlib/Measurements/Three-Phase V-I Measurement  VoltageMeasurement=phase-to-ground  SetLabelV=off  LabelV=Vabc  Vpu=off  VpuLL=off  CurrentMeasurement=yes  SetLabelI=off  LabelI=Iabc  Ipu=off  Pbase=100e6  Vbase=500e3  OutputType=Complex  PhasorSimulation=off  PSBequivalent=0
  UIptg_35 : Scope  NumInputPorts=2
  Uptg_35 : Display
      settings: Format=bank
  a : PMIOPort  Side=Right
  b : PMIOPort  Port=2  Side=Right
  c : PMIOPort  Port=3  Side=Right
  A : PMIOPort  Port=4  Side=Left
  B : PMIOPort  Port=5  Side=Left
  C : PMIOPort  Port=6  Side=Left
  tag scope: I_ptg_35=global, P_ptg_35=global, Q_ptg_35=global, S_ptg_35=global, U_ptg_35=global
  wires:
  S/1 -> [S_ptg_35]
  Real-Ima to Complex/1 -> S/1
  [S_ptg_35] -> Sptg_35/1
  [S_ptg_35] -> SSptg_35/1
  [P_ptg_35] -> RMSpt_35/1
  RMSpt_35/1 -> Pptg_35/1
  RMS35/1 -> Qptg_35/1
  [U_ptg_35] -> RMS3/1
  RMS3/1 -> Uptg_35/1
  [P_ptg_35] -> Real-Ima to Complex/1
  [Q_ptg_35] -> RMS35/1
  [I_ptg_35] -> RMS4/1
  RMS4/1 -> Iptg_35/1
  [U_ptg_35] -> UIptg_35/1  "U"
  [P_ptg_35] -> PQptg_35/1  "P"
  [I_ptg_35] -> UIptg_35/2  "I"
  Three-Phase V-I Measurementpt_35/1 -> [U_ptg_35]
  [Q_ptg_35] -> Real-Ima to Complex/2
  Three-Phase V-I Measurementpt_35/2 -> [I_ptg_35]
  [U_ptg_35] -> "Power0 (3ph, Instantaneous)"/1
  [I_ptg_35] -> "Power0 (3ph, Instantaneous)"/2
  "Power0 (3ph, Instantaneous)"/2 -> [Q_ptg_35]
  "Power0 (3ph, Instantaneous)"/1 -> [P_ptg_35]
  [Q_ptg_35] -> PQptg_35/2  "Q"
  connections:
  Three-Phase V-I Measurementpt_35/LConn1 -- A/RConn1
  Three-Phase V-I Measurementpt_35/RConn1 -- a/RConn1
  Three-Phase V-I Measurementpt_35/LConn2 -- B/RConn1
  Three-Phase V-I Measurementpt_35/LConn3 -- C/RConn1
  Three-Phase V-I Measurementpt_35/RConn3 -- c/RConn1
  Three-Phase V-I Measurementpt_35/RConn2 -- b/RConn1

== system RADTRANS002/M_IN_Город_4_1 ==
  Iptg_41 : Display
      settings: Format=bank
  PQptg_41 : Scope  NumInputPorts=2
  "Power0 (3ph, Instantaneous)" : powerlib_meascontrol/Measurements/Power (3ph, Instantaneous)
  Pptg_41 : Display
      settings: Format=bank
  Qptg_41 : Display
      settings: Format=bank
  RMS3 : dspstat3/RMS  run=off  directionMode=Each column  dimension=1  InputProcessing=Columns as channels (frame based)  reset_popup=None
  RMS4 : dspstat3/RMS  run=off  directionMode=Each column  dimension=1  InputProcessing=Columns as channels (frame based)  reset_popup=None
  RMS41 : dspstat3/RMS  run=off  directionMode=Each column  dimension=1  InputProcessing=Columns as channels (frame based)  reset_popup=None
  RMSpt_41 : dspstat3/RMS  run=off  directionMode=Each column  dimension=1  InputProcessing=Columns as channels (frame based)  reset_popup=None
  Real-Ima to Complex : RealImagToComplex
  S : Abs
  SSptg_41 : Scope
  Sptg_41 : Display
      settings: Format=bank
  Three-Phase V-I Measurementpt_41 : powerlib/Measurements/Three-Phase V-I Measurement  VoltageMeasurement=phase-to-ground  SetLabelV=off  LabelV=Vabc  Vpu=off  VpuLL=off  CurrentMeasurement=yes  SetLabelI=off  LabelI=Iabc  Ipu=off  Pbase=100e6  Vbase=500e3  OutputType=Complex  PhasorSimulation=off  PSBequivalent=0
  UIptg_41 : Scope  NumInputPorts=2
  Uptg_41 : Display
      settings: Format=bank
  a : PMIOPort  Side=Right
  b : PMIOPort  Port=2  Side=Right
  c : PMIOPort  Port=3  Side=Right
  A : PMIOPort  Port=4  Side=Left
  B : PMIOPort  Port=5  Side=Left
  C : PMIOPort  Port=6  Side=Left
  tag scope: I_ptg_41=global, P_ptg_41=global, Q_ptg_41=global, S_ptg_41=global, U_ptg_41=global
  wires:
  S/1 -> [S_ptg_41]
  Real-Ima to Complex/1 -> S/1
  [S_ptg_41] -> Sptg_41/1
  [S_ptg_41] -> SSptg_41/1
  [P_ptg_41] -> RMSpt_41/1
  RMSpt_41/1 -> Pptg_41/1
  RMS41/1 -> Qptg_41/1
  [U_ptg_41] -> RMS3/1
  RMS3/1 -> Uptg_41/1
  [P_ptg_41] -> Real-Ima to Complex/1
  [Q_ptg_41] -> RMS41/1
  [I_ptg_41] -> RMS4/1
  RMS4/1 -> Iptg_41/1
  [U_ptg_41] -> UIptg_41/1  "U"
  [P_ptg_41] -> PQptg_41/1  "P"
  [I_ptg_41] -> UIptg_41/2  "I"
  Three-Phase V-I Measurementpt_41/1 -> [U_ptg_41]
  [Q_ptg_41] -> Real-Ima to Complex/2
  Three-Phase V-I Measurementpt_41/2 -> [I_ptg_41]
  [U_ptg_41] -> "Power0 (3ph, Instantaneous)"/1
  [I_ptg_41] -> "Power0 (3ph, Instantaneous)"/2
  "Power0 (3ph, Instantaneous)"/2 -> [Q_ptg_41]
  "Power0 (3ph, Instantaneous)"/1 -> [P_ptg_41]
  [Q_ptg_41] -> PQptg_41/2  "Q"
  connections:
  Three-Phase V-I Measurementpt_41/LConn1 -- A/RConn1
  Three-Phase V-I Measurementpt_41/RConn1 -- a/RConn1
  Three-Phase V-I Measurementpt_41/LConn2 -- B/RConn1
  Three-Phase V-I Measurementpt_41/LConn3 -- C/RConn1
  Three-Phase V-I Measurementpt_41/RConn3 -- c/RConn1
  Three-Phase V-I Measurementpt_41/RConn2 -- b/RConn1

== system RADTRANS002/M_IN_Город_4_2 ==
  Iptg_43 : Display
      settings: Format=bank
  PQptg_43 : Scope  NumInputPorts=2
  "Power0 (3ph, Instantaneous)" : powerlib_meascontrol/Measurements/Power (3ph, Instantaneous)
  Pptg_43 : Display
      settings: Format=bank
  Qptg_43 : Display
      settings: Format=bank
  RMS3 : dspstat3/RMS  run=off  directionMode=Each column  dimension=1  InputProcessing=Columns as channels (frame based)  reset_popup=None
  RMS4 : dspstat3/RMS  run=off  directionMode=Each column  dimension=1  InputProcessing=Columns as channels (frame based)  reset_popup=None
  RMS43 : dspstat3/RMS  run=off  directionMode=Each column  dimension=1  InputProcessing=Columns as channels (frame based)  reset_popup=None
  RMSpt_43 : dspstat3/RMS  run=off  directionMode=Each column  dimension=1  InputProcessing=Columns as channels (frame based)  reset_popup=None
  Real-Ima to Complex : RealImagToComplex
  S : Abs
  SSptg_43 : Scope
  Sptg_43 : Display
      settings: Format=bank
  Three-Phase V-I Measurementpt_43 : powerlib/Measurements/Three-Phase V-I Measurement  VoltageMeasurement=phase-to-ground  SetLabelV=off  LabelV=Vabc  Vpu=off  VpuLL=off  CurrentMeasurement=yes  SetLabelI=off  LabelI=Iabc  Ipu=off  Pbase=100e6  Vbase=500e3  OutputType=Complex  PhasorSimulation=off  PSBequivalent=0
  UIptg_43 : Scope  NumInputPorts=2
  Uptg_43 : Display
      settings: Format=bank
  a : PMIOPort  Side=Right
  b : PMIOPort  Port=2  Side=Right
  c : PMIOPort  Port=3  Side=Right
  A : PMIOPort  Port=4  Side=Left
  B : PMIOPort  Port=5  Side=Left
  C : PMIOPort  Port=6  Side=Left
  tag scope: I_ptg_43=global, P_ptg_43=global, Q_ptg_43=global, S_ptg_43=global, U_ptg_43=global
  wires:
  S/1 -> [S_ptg_43]
  Real-Ima to Complex/1 -> S/1
  [S_ptg_43] -> Sptg_43/1
  [S_ptg_43] -> SSptg_43/1
  [P_ptg_43] -> RMSpt_43/1
  RMSpt_43/1 -> Pptg_43/1
  RMS43/1 -> Qptg_43/1
  [U_ptg_43] -> RMS3/1
  RMS3/1 -> Uptg_43/1
  [P_ptg_43] -> Real-Ima to Complex/1
  [Q_ptg_43] -> RMS43/1
  [I_ptg_43] -> RMS4/1
  RMS4/1 -> Iptg_43/1
  [U_ptg_43] -> UIptg_43/1  "U"
  [P_ptg_43] -> PQptg_43/1  "P"
  [I_ptg_43] -> UIptg_43/2  "I"
  Three-Phase V-I Measurementpt_43/1 -> [U_ptg_43]
  [Q_ptg_43] -> Real-Ima to Complex/2
  Three-Phase V-I Measurementpt_43/2 -> [I_ptg_43]
  [U_ptg_43] -> "Power0 (3ph, Instantaneous)"/1
  [I_ptg_43] -> "Power0 (3ph, Instantaneous)"/2
  "Power0 (3ph, Instantaneous)"/2 -> [Q_ptg_43]
  "Power0 (3ph, Instantaneous)"/1 -> [P_ptg_43]
  [Q_ptg_43] -> PQptg_43/2  "Q"
  connections:
  Three-Phase V-I Measurementpt_43/LConn1 -- A/RConn1
  Three-Phase V-I Measurementpt_43/RConn1 -- a/RConn1
  Three-Phase V-I Measurementpt_43/LConn2 -- B/RConn1
  Three-Phase V-I Measurementpt_43/LConn3 -- C/RConn1
  Three-Phase V-I Measurementpt_43/RConn3 -- c/RConn1
  Three-Phase V-I Measurementpt_43/RConn2 -- b/RConn1

== system RADTRANS002/M_IN_Город_4_3 ==
  Iptg_45 : Display
      settings: Format=bank
  PQptg_45 : Scope  NumInputPorts=2
  "Power0 (3ph, Instantaneous)" : powerlib_meascontrol/Measurements/Power (3ph, Instantaneous)
  Pptg_45 : Display
      settings: Format=bank
  Qptg_45 : Display
      settings: Format=bank
  RMS3 : dspstat3/RMS  run=off  directionMode=Each column  dimension=1  InputProcessing=Columns as channels (frame based)  reset_popup=None
  RMS4 : dspstat3/RMS  run=off  directionMode=Each column  dimension=1  InputProcessing=Columns as channels (frame based)  reset_popup=None
  RMS45 : dspstat3/RMS  run=off  directionMode=Each column  dimension=1  InputProcessing=Columns as channels (frame based)  reset_popup=None
  RMSpt_45 : dspstat3/RMS  run=off  directionMode=Each column  dimension=1  InputProcessing=Columns as channels (frame based)  reset_popup=None
  Real-Ima to Complex : RealImagToComplex
  S : Abs
  SSptg_45 : Scope
  Sptg_45 : Display
      settings: Format=bank
  Three-Phase V-I Measurementpt_45 : powerlib/Measurements/Three-Phase V-I Measurement  VoltageMeasurement=phase-to-ground  SetLabelV=off  LabelV=Vabc  Vpu=off  VpuLL=off  CurrentMeasurement=yes  SetLabelI=off  LabelI=Iabc  Ipu=off  Pbase=100e6  Vbase=500e3  OutputType=Complex  PhasorSimulation=off  PSBequivalent=0
  UIptg_45 : Scope  NumInputPorts=2
  Uptg_45 : Display
      settings: Format=bank
  a : PMIOPort  Side=Right
  b : PMIOPort  Port=2  Side=Right
  c : PMIOPort  Port=3  Side=Right
  A : PMIOPort  Port=4  Side=Left
  B : PMIOPort  Port=5  Side=Left
  C : PMIOPort  Port=6  Side=Left
  tag scope: I_ptg_45=global, P_ptg_45=global, Q_ptg_45=global, S_ptg_45=global, U_ptg_45=global
  wires:
  S/1 -> [S_ptg_45]
  Real-Ima to Complex/1 -> S/1
  [S_ptg_45] -> Sptg_45/1
  [S_ptg_45] -> SSptg_45/1
  [P_ptg_45] -> RMSpt_45/1
  RMSpt_45/1 -> Pptg_45/1
  RMS45/1 -> Qptg_45/1
  [U_ptg_45] -> RMS3/1
  RMS3/1 -> Uptg_45/1
  [P_ptg_45] -> Real-Ima to Complex/1
  [Q_ptg_45] -> RMS45/1
  [I_ptg_45] -> RMS4/1
  RMS4/1 -> Iptg_45/1
  [U_ptg_45] -> UIptg_45/1  "U"
  [P_ptg_45] -> PQptg_45/1  "P"
  [I_ptg_45] -> UIptg_45/2  "I"
  Three-Phase V-I Measurementpt_45/1 -> [U_ptg_45]
  [Q_ptg_45] -> Real-Ima to Complex/2
  Three-Phase V-I Measurementpt_45/2 -> [I_ptg_45]
  [U_ptg_45] -> "Power0 (3ph, Instantaneous)"/1
  [I_ptg_45] -> "Power0 (3ph, Instantaneous)"/2
  "Power0 (3ph, Instantaneous)"/2 -> [Q_ptg_45]
  "Power0 (3ph, Instantaneous)"/1 -> [P_ptg_45]
  [Q_ptg_45] -> PQptg_45/2  "Q"
  connections:
  Three-Phase V-I Measurementpt_45/LConn1 -- A/RConn1
  Three-Phase V-I Measurementpt_45/RConn1 -- a/RConn1
  Three-Phase V-I Measurementpt_45/LConn2 -- B/RConn1
  Three-Phase V-I Measurementpt_45/LConn3 -- C/RConn1
  Three-Phase V-I Measurementpt_45/RConn3 -- c/RConn1
  Three-Phase V-I Measurementpt_45/RConn2 -- b/RConn1

== system RADTRANS002/M_IN_Город_4_4 ==
  Iptg_47 : Display
      settings: Format=bank
  PQptg_47 : Scope  NumInputPorts=2
  "Power0 (3ph, Instantaneous)" : powerlib_meascontrol/Measurements/Power (3ph, Instantaneous)
  Pptg_47 : Display
      settings: Format=bank
  Qptg_47 : Display
      settings: Format=bank
  RMS3 : dspstat3/RMS  run=off  directionMode=Each column  dimension=1  InputProcessing=Columns as channels (frame based)  reset_popup=None
  RMS4 : dspstat3/RMS  run=off  directionMode=Each column  dimension=1  InputProcessing=Columns as channels (frame based)  reset_popup=None
  RMS47 : dspstat3/RMS  run=off  directionMode=Each column  dimension=1  InputProcessing=Columns as channels (frame based)  reset_popup=None
  RMSpt_47 : dspstat3/RMS  run=off  directionMode=Each column  dimension=1  InputProcessing=Columns as channels (frame based)  reset_popup=None
  Real-Ima to Complex : RealImagToComplex
  S : Abs
  SSptg_47 : Scope
  Sptg_47 : Display
      settings: Format=bank
  Three-Phase V-I Measurementpt_47 : powerlib/Measurements/Three-Phase V-I Measurement  VoltageMeasurement=phase-to-ground  SetLabelV=off  LabelV=Vabc  Vpu=off  VpuLL=off  CurrentMeasurement=yes  SetLabelI=off  LabelI=Iabc  Ipu=off  Pbase=100e6  Vbase=500e3  OutputType=Complex  PhasorSimulation=off  PSBequivalent=0
  UIptg_47 : Scope  NumInputPorts=2
  Uptg_47 : Display
      settings: Format=bank
  a : PMIOPort  Side=Right
  b : PMIOPort  Port=2  Side=Right
  c : PMIOPort  Port=3  Side=Right
  A : PMIOPort  Port=4  Side=Left
  B : PMIOPort  Port=5  Side=Left
  C : PMIOPort  Port=6  Side=Left
  tag scope: I_ptg_47=global, P_ptg_47=global, Q_ptg_47=global, S_ptg_47=global, U_ptg_47=global
  wires:
  S/1 -> [S_ptg_47]
  Real-Ima to Complex/1 -> S/1
  [S_ptg_47] -> Sptg_47/1
  [S_ptg_47] -> SSptg_47/1
  [P_ptg_47] -> RMSpt_47/1
  RMSpt_47/1 -> Pptg_47/1
  RMS47/1 -> Qptg_47/1
  [U_ptg_47] -> RMS3/1
  RMS3/1 -> Uptg_47/1
  [P_ptg_47] -> Real-Ima to Complex/1
  [Q_ptg_47] -> RMS47/1
  [I_ptg_47] -> RMS4/1
  RMS4/1 -> Iptg_47/1
  [U_ptg_47] -> UIptg_47/1  "U"
  [P_ptg_47] -> PQptg_47/1  "P"
  [I_ptg_47] -> UIptg_47/2  "I"
  Three-Phase V-I Measurementpt_47/1 -> [U_ptg_47]
  [Q_ptg_47] -> Real-Ima to Complex/2
  Three-Phase V-I Measurementpt_47/2 -> [I_ptg_47]
  [U_ptg_47] -> "Power0 (3ph, Instantaneous)"/1
  [I_ptg_47] -> "Power0 (3ph, Instantaneous)"/2
  "Power0 (3ph, Instantaneous)"/2 -> [Q_ptg_47]
  "Power0 (3ph, Instantaneous)"/1 -> [P_ptg_47]
  [Q_ptg_47] -> PQptg_47/2  "Q"
  connections:
  Three-Phase V-I Measurementpt_47/LConn1 -- A/RConn1
  Three-Phase V-I Measurementpt_47/RConn1 -- a/RConn1
  Three-Phase V-I Measurementpt_47/LConn2 -- B/RConn1
  Three-Phase V-I Measurementpt_47/LConn3 -- C/RConn1
  Three-Phase V-I Measurementpt_47/RConn3 -- c/RConn1
  Three-Phase V-I Measurementpt_47/RConn2 -- b/RConn1

== system RADTRANS002/M_IN_Город_5_1 ==
  Iptg_53 : Display
      settings: Format=bank
  PQptg_53 : Scope  NumInputPorts=2
  "Power0 (3ph, Instantaneous)" : powerlib_meascontrol/Measurements/Power (3ph, Instantaneous)
  Pptg_53 : Display
      settings: Format=bank
  Qptg_53 : Display
      settings: Format=bank
  RMS3 : dspstat3/RMS  run=off  directionMode=Each column  dimension=1  InputProcessing=Columns as channels (frame based)  reset_popup=None
  RMS4 : dspstat3/RMS  run=off  directionMode=Each column  dimension=1  InputProcessing=Columns as channels (frame based)  reset_popup=None
  RMS53 : dspstat3/RMS  run=off  directionMode=Each column  dimension=1  InputProcessing=Columns as channels (frame based)  reset_popup=None
  RMSpt_53 : dspstat3/RMS  run=off  directionMode=Each column  dimension=1  InputProcessing=Columns as channels (frame based)  reset_popup=None
  Real-Ima to Complex : RealImagToComplex
  S : Abs
  SSptg_53 : Scope
  Sptg_53 : Display
      settings: Format=bank
  Three-Phase V-I Measurementpt_53 : powerlib/Measurements/Three-Phase V-I Measurement  VoltageMeasurement=phase-to-ground  SetLabelV=off  LabelV=Vabc  Vpu=off  VpuLL=off  CurrentMeasurement=yes  SetLabelI=off  LabelI=Iabc  Ipu=off  Pbase=100e6  Vbase=500e3  OutputType=Complex  PhasorSimulation=off  PSBequivalent=0
  UIptg_53 : Scope  NumInputPorts=2
  Uptg_53 : Display
      settings: Format=bank
  a : PMIOPort  Side=Right
  b : PMIOPort  Port=2  Side=Right
  c : PMIOPort  Port=3  Side=Right
  A : PMIOPort  Port=4  Side=Left
  B : PMIOPort  Port=5  Side=Left
  C : PMIOPort  Port=6  Side=Left
  tag scope: I_ptg_53=global, P_ptg_53=global, Q_ptg_53=global, S_ptg_53=global, U_ptg_53=global
  wires:
  S/1 -> [S_ptg_53]
  Real-Ima to Complex/1 -> S/1
  [S_ptg_53] -> Sptg_53/1
  [S_ptg_53] -> SSptg_53/1
  [P_ptg_53] -> RMSpt_53/1
  RMSpt_53/1 -> Pptg_53/1
  RMS53/1 -> Qptg_53/1
  [U_ptg_53] -> RMS3/1
  RMS3/1 -> Uptg_53/1
  [P_ptg_53] -> Real-Ima to Complex/1
  [Q_ptg_53] -> RMS53/1
  [I_ptg_53] -> RMS4/1
  RMS4/1 -> Iptg_53/1
  [U_ptg_53] -> UIptg_53/1  "U"
  [P_ptg_53] -> PQptg_53/1  "P"
  [I_ptg_53] -> UIptg_53/2  "I"
  Three-Phase V-I Measurementpt_53/1 -> [U_ptg_53]
  [Q_ptg_53] -> Real-Ima to Complex/2
  Three-Phase V-I Measurementpt_53/2 -> [I_ptg_53]
  [U_ptg_53] -> "Power0 (3ph, Instantaneous)"/1
  [I_ptg_53] -> "Power0 (3ph, Instantaneous)"/2
  "Power0 (3ph, Instantaneous)"/2 -> [Q_ptg_53]
  "Power0 (3ph, Instantaneous)"/1 -> [P_ptg_53]
  [Q_ptg_53] -> PQptg_53/2  "Q"
  connections:
  Three-Phase V-I Measurementpt_53/LConn1 -- A/RConn1
  Three-Phase V-I Measurementpt_53/RConn1 -- a/RConn1
  Three-Phase V-I Measurementpt_53/LConn2 -- B/RConn1
  Three-Phase V-I Measurementpt_53/LConn3 -- C/RConn1
  Three-Phase V-I Measurementpt_53/RConn3 -- c/RConn1
  Three-Phase V-I Measurementpt_53/RConn2 -- b/RConn1
